simulink model "Example"  (R2023b)
settings: Solver=FixedStepDiscrete  StartTime=0.0  StopTime=0.1  FixedStep=0.01  RelTol=1e-3  EnableMultiTasking=on
values from neighbouring files (symbols this model uses):
  Aps_val1 = 60    [Test_Param.m]
  Aps_val2 = 40    [Test_Param.m]
  Aps_val3 = 20    [Test_Param.m]
  Default_Value = 5    [Test_Param.m]
  Gear_Val1 = 4    [Test_Param.m]
  Gear_Val2 = 3    [Test_Param.m]
  Gear_Val3 = 2    [Test_Param.m]
  Gear_Val4 = 1    [Test_Param.m]
  vsp_val = 50    [Test_Param.m]
settings Model: Creator=The MathWorks, Inc.  LastModifiedBy=22011083
settings SolverCC: AlgebraicLoopSolver=TrustRegion
settings DataIOCC: LimitDataPoints=on  SaveFormat=Array  ReturnWorkspaceOutputs=off
settings OptimizationCC: ConditionallyExecuteInputs=off  DefaultParameterBehavior=Inlined  InlineInvariantSignals=on  ExpressionDepthLimit=2147483647  InitFltsAndDblsToZero=on  EfficientMapNaN2IntZero=off  LifeSpan=inf
settings DebuggingCC: SaveWithParameterizedLinksMsg=none  MergeDetectMultiDrivingBlocksExec=none  SignalResolutionControl=TryResolveAllWithWarning  SolverPrmCheckMsg=warning  FcnCallInpInsideContextMsg=warning  UnconnectedInputMsg=warning  UnconnectedOutputMsg=warning  UnconnectedLineMsg=warning  AllowSymbolicDim=off  StateNameClashWarn=warning  SFUnexpectedBacktrackingDiag=warning  SFNoUnconditionalDefaultTransitionDiag=warning  SFExecutionAtInitializationDiag=none  ArithmeticOperatorsInVariantConditions=warning
settings HardwareCC: ProdBitPerPointer=32  ProdBitPerSizeT=32  ProdBitPerPtrDiffT=32  ProdLargestAtomicFloat=None  ProdIntDivRoundTo=Undefined  ProdEndianess=Unspecified  ProdWordSize=32  ProdHWDeviceType=32-bit Generic
settings ModelReferenceCC: EnableRefExpFcnMdlSchedulingChecks=on  PropagateSignalLabelsOutOfModel=off
settings SFSimCC: SimUseLocalCustomCode=off  CustomCodeUndefinedFunction=UseInterfaceOnly
settings RTWCC: GenCodeOnly=on  RTWUseLocalCustomCode=off  DLArmComputeVersion=19.05
settings CodeAppCC: StateflowObjectComments=on
settings GRTTargetCC: TargetFcnLib=ansi_tfl_tmw.mat  TargetLangStandard=C89/C90 (ANSI)  CombineOutputUpdateFcns=off  GRTInterface=on
settings ConfigComp: CovMetricSettings=dcme  CovHTMLOptions=-sRT=1 -sVT=0 -aTS=1 -agT=1 -bRG=1 -bTC=1 -hTR=0 -nFC=0 -nFD=0 -scm=1 -bcm=1 -xEv=0 -xEM=0 -req=1  CovEnableCumulative=off  CovCumulativeReport=on  DVMakeOutputFilesUnique=off  DVParameterConfiguration=UseParameterConfigFile  DVParameters=on  DVModelCoverageObjectives=MCDC  DVMaxTestCaseSteps=500  DVTestSuiteOptimization=Auto  DVAssertions=EnableAll  DVProofAssumptions=EnableAll  DVDetectActiveLogic=on  DVProvingStrategy=FindViolation  DVReduceRationalApprox=off

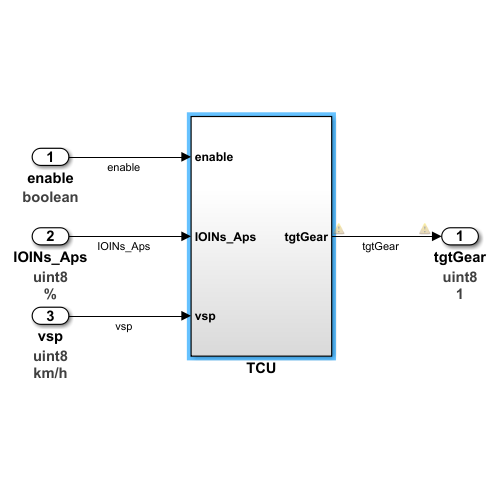
[thumbnail: Simulink's stored preview of the top-level diagram]
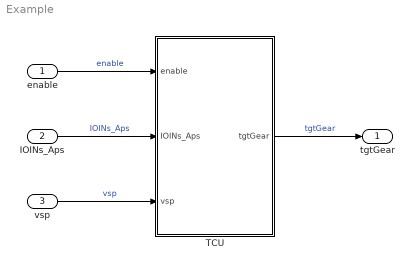
== system Example ==
  enable : Inport  OutDataTypeStr=boolean
      settings: AttributesFormatString=%<OutDataTypeStr>
  IOINs_Aps : Inport  Port=2  OutDataTypeStr=uint8  Unit=%
      settings: AttributesFormatString=|
      | %<OutDataTypeStr>
      | %<Unit>
  vsp : Inport  Port=3  OutDataTypeStr=uint8  Unit=km/h
      settings: AttributesFormatString=|
      | %<OutDataTypeStr>
      | %<Unit>
  TCU : Subsystem
  tgtGear : Outport  OutDataTypeStr=uint8  Unit=1  VectorParamsAs1DForOutWhenUnconnected=off
      settings: AttributesFormatString=|
      | %<OutDataTypeStr>
      | %<Unit>
  wires:
  enable/1 -> TCU/1(enable)  "enable"
  IOINs_Aps/1 -> TCU/2(IOINs_Aps)  "IOINs_Aps"
  vsp/1 -> TCU/3(vsp)  "vsp"
  TCU/1(tgtGear) -> tgtGear/1  "tgtGear"

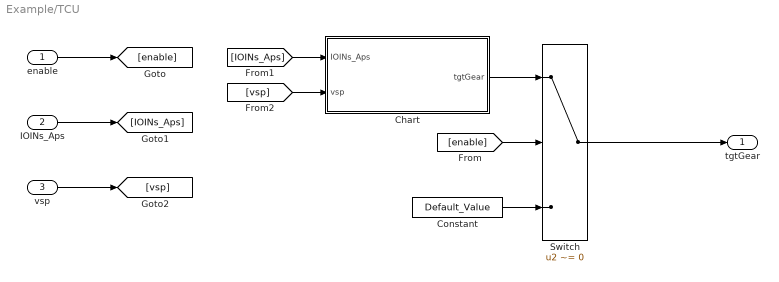
== system Example/TCU ==
  enable : Inport  OutDataTypeStr=boolean
      settings: AttributesFormatString=%<OutDataTypeStr>
  IOINs_Aps : Inport  Port=2  OutDataTypeStr=uint8  Unit=%
      settings: AttributesFormatString=|
      | %<OutDataTypeStr>
      | %<Unit>
  vsp : Inport  Port=3  OutDataTypeStr=uint8  Unit=km/h
      settings: AttributesFormatString=|
      | %<OutDataTypeStr>
      | %<Unit>
  Chart : Stateflow chart  TreatAsAtomicUnit=on
  Constant : Constant  Value=Default_Value
  Switch : Switch  Criteria=u2 ~= 0  OutDataTypeStr=uint8  RndMeth=Simplest  InputSameDT=off
      settings: AttributesFormatString=%<OutDataTypeStr>
  tgtGear : Outport  OutDataTypeStr=uint8  Unit=1  VectorParamsAs1DForOutWhenUnconnected=off
      settings: AttributesFormatString=|
      | %<OutDataTypeStr>
      | %<Unit>
  wires:
  IOINs_Aps/1 -> [IOINs_Aps]
  enable/1 -> [enable]
  vsp/1 -> [vsp]
  Switch/1 -> tgtGear/1
  [enable] -> Switch/2
  Constant/1 -> Switch/3
  Chart/1(tgtGear) -> Switch/1
  [vsp] -> Chart/2(vsp)
  [IOINs_Aps] -> Chart/1(IOINs_Aps)

== stateflow chart Example/TCU/Chart ==
  state GearSel [function]
    (default) -> (junction 75)
    (junction 75) -> (junction 76) [order 1] : [IOINs_Aps >= Aps_val1] {tgtGear = Gear_Val1;}
    (junction 75) -> (junction 78) [order 2]
    (junction 76) -> (junction 77)
    (junction 78) -> (junction 77) [order 1] : [IOINs_Aps >= Aps_val2] {tgtGear = Gear_Val2;}
    (junction 78) -> (junction 86) [order 2]
    (junction 77) -> (junction 87)
    (junction 86) -> (junction 87) [order 1] : [IOINs_Aps >= Aps_val3] {tgtGear = Gear_Val3;}
    (junction 86) -> (junction 92) [order 2]
    (junction 87) -> (junction 91)
    (junction 92) -> (junction 91) : {tgtGear = Gear_Val4;}
  (default) -> (junction 61) : {tgtGear = 0;}
  (junction 61) -> (junction 65) [order 1] : [vsp >= vsp_val] {GearSel();}
  (junction 61) -> (junction 83) [order 2]
  (junction 65) -> (junction 84)
  (junction 83) -> (junction 84) : % Hold
  data: tgtGear output uint8; IOINs_Aps input uint8; vsp input uint8; vsp_val parameter; Aps_val1 parameter; Aps_val2 parameter; Aps_val3 parameter; Gear_Val1 parameter; Gear_Val2 parameter; Gear_Val3 parameter; Gear_Val4 parameter
